simulink model "PSK_1"  (R2017b)
settings: Solver=VariableStepAuto  StartTime=0.0  StopTime=10.0  MaxStep=0.01  MinStep=0.001  RelTol=1e-3
libraries: dsparch4 x1
settings Model: Creator=ayadd  LastModifiedBy=ayadd
settings SolverCC: ShapePreserveControl=EnableAll  ZeroCrossAlgorithm=Adaptive

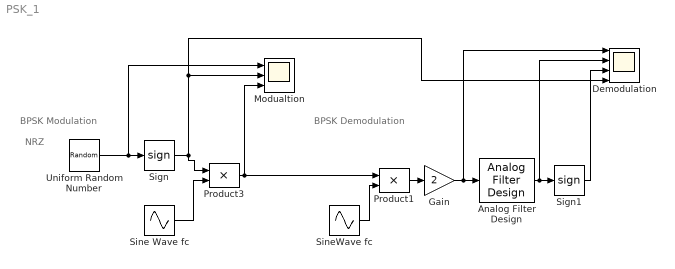
== system PSK_1 ==
  note: NRZ
  note: BPSK Demodulation
  note: BPSK Modulation
  Analog Filter Design : dsparch4/Analog Filter Design  method=Butterworth  filttype=Lowpass  N=8  Wlo=10*2*pi  Whi=80  Rp=2  Rs=40
  Demodulation : Scope  NumInputPorts=4
  Gain : Gain  Gain=2
  Modualtion : Scope  NumInputPorts=3
  Product1 : Product  SaturateOnIntegerOverflow=on  InputSameDT=on  OutDataTypeStr=Inherit: Same as first input
  Product3 : Product  SaturateOnIntegerOverflow=on  InputSameDT=on  OutDataTypeStr=Inherit: Same as first input
  Sign : Signum
  Sign1 : Signum
  Sine Wave fc : Sin  Frequency=4*2*pi  SampleTime=0
  SineWave fc : Sin  Frequency=4*2*pi  SampleTime=0
  Uniform Random Number : UniformRandomNumber  SampleTime=1
  wires:
  Uniform Random Number/1 -> Sign/1, Modualtion/1
  Product1/1 -> Gain/1
  Analog Filter Design/1 -> Demodulation/2, Sign1/1
  Gain/1 -> Demodulation/1, Analog Filter Design/1
  Sign/1 -> Product3/1, Demodulation/4, Modualtion/2
  SineWave fc/1 -> Product1/2
  Product3/1 -> Modualtion/3, Product1/1
  Sign1/1 -> Demodulation/3
  Sine Wave fc/1 -> Product3/2
